simulink model "ur_ros"  (R2024a)
settings: Solver=FixedStepAuto  StartTime=0.0  StopTime=inf  RelTol=1e-3
undefined symbols (not defined in the file): duration, effort, index, joint1, joint2, joint3, joint4, joint5, joint6, joint_name, model_name, q0, Ts, ur
libraries: robotgazebolib x26, robotmaniplib x3, slpidlib x1
settings Model: Creator=26092  LastModifiedBy=26092

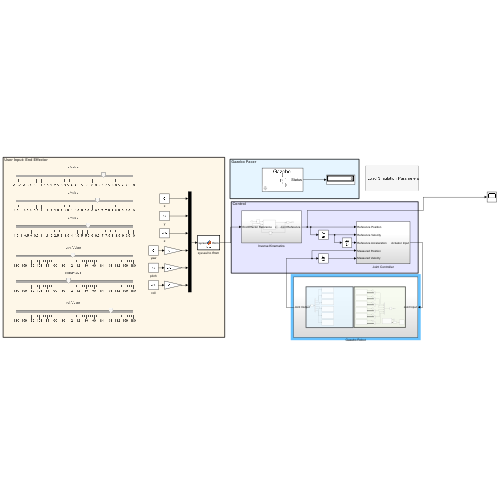
[thumbnail: Simulink's stored preview of the top-level diagram]
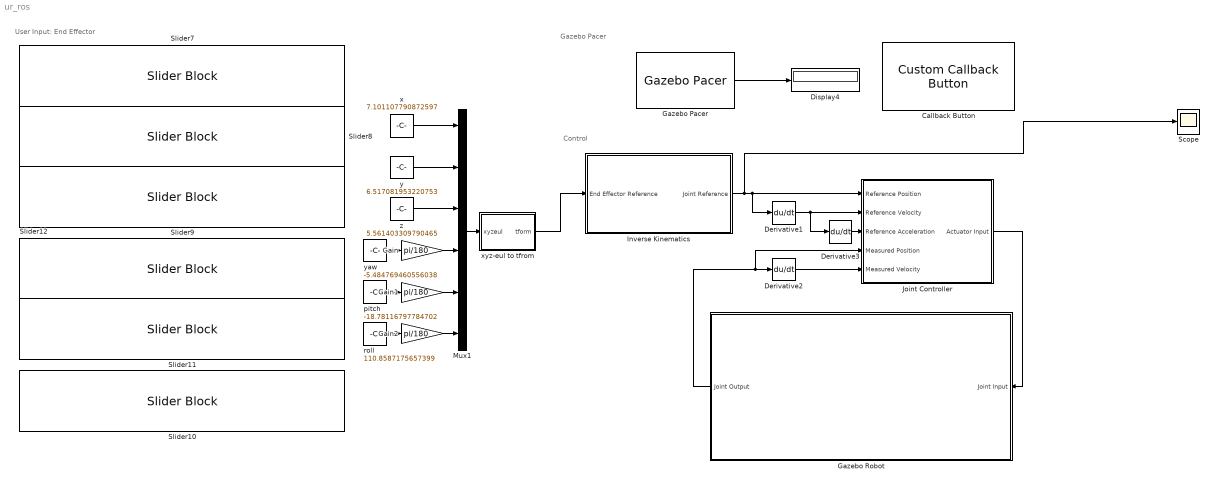
== system ur_ros ==
  note: User Input: End Effector
  note: Control
  note: Gazebo Pacer
  Callback Button : CustomCallbackButton  Configuration="{\"components\":[{\"name\":\"BackgroundImageComponent\",\"settings\":{\"image\":{\"size\":[0,0],\"src\":\"default\",\"srcOrientation\":\"Right\"},\"position\":[0,0,1,1]}},{\"name\":\"ButtonStateComponent\",\"settings\":{\"buttonType\":\"momentary\",\"clickFcn\":\" % Set sample times\\n  Ts = 0.01;\\n  Ts_trajectory = 0.05;\\n\\n  % Load the robot - 使用自定义URDF模型\\n  robot = importrobot('ur.urdf');\\n  robot.Gravity = [0 0 -9.81];\\n  robot.DataFormat = 'column';\\n\\n  % 显示机器人信息确认加载\\n  showdetails(robot);\\n  disp('机器人模型 robot 已成功加载！');\\n\\n  % IK initial guess\\n  q0 = [0 -70 140 0 0 0]' * pi\\/180;\\n\\n  % Custom bus objects\\n  load('custom_busobjects_basic');\",\"onValue\":1,\"position\":[0,0,1,1],\"pressDelay\":\"500\",\"pressFcn\":\"\",\"repeatInterval\":\"0\",\"states\":[{\"horizontalAlignment\":\"center\",\"image\":{\"position\":[0,0,1,1],\"size\":[1,1],\"src\":\"default\",\"srcOrientation\":\"Right\"},\"label\":{\"color\":[0.01176470588,0.01176470588,0.01176470588,1],\"icon\":{\"size\":[0,0],\"src\":\"default\",\"srcOrientation\":\"Right\"},\"iconPlacement\":\"left\",\"opacity\":1,\"show\":true,\"text\":{\"content\":\"Load Simulation Parameters\",\"font\":\"Helvetica\",\"fontSize\":15}},\"labelOffset\":[0,0],\"verticalAlignment\":\"middle\"},{\"horizontalAlignment\":\"center\",\"image\":{\"position\":[0,0,1,1],\"size\":[1,1],\"src\":\"default\",\"srcOrientation\":\"Right\"},\"label\":{\"color\":[0.01176470588,0.01176470588,0.01176470588,1],\"icon\":{\"size\":[0,0],\"src\":\"default\",\"srcOrientation\":\"Right\"},\"iconPlacement\":\"left\",\"opacity\":1,\"show\":true,\"text\":{\"content\":\"Load Simulation Parameters\",\"font\":\"Helvetica\",\"fontSize\":15}},\"labelOffset\":[0,0],\"verticalAlignment\":\"middle\"},{\"horizontalAlignment\":\"center\",\"image\":{\"position\":[0,0,1,1],\"size\":[1,1],\"src\":\"default\",\"srcOrientation\":\"Right\"},\"label\":{\"color\":[0.01176470588,0.01176470588,0.01176470588,1],\"icon\":{\"size\":[0,0],\"src\":\"default\",\"srcOrientation\":\"Right\"},\"iconPlacement\":\"left\",\"opacity\":1,\"show\":true,\"text\":{\"content\":\"Load Simulation Parameters\",\"font\":\"Helvetica\",\"fontSize\":15}},\"labelOffset\":[0,0],\"verticalAlignment\":\"middle\"},{\"horizontalAlignment\":\"center\",\"image\":{\"position\":[0,0,1,1],\"size\":[1,1],\"src\":\"default\",\"srcOrientation\":\"Right\"},\"label\":{\"color\":[0.01176470588,0.01176470588,0.01176470588,1],\"icon\":{\"size\":[0,0],\"src\":\"default\",\"srcOrientation\":\"Right\"},\"iconPlacement\":\"left\",\"opacity\":1,\"show\":true,\"text\":{\"content\":\"Load Simulation Parameters\",\"font\":\"Helvetica\",\"fontSize\":15}},\"labelOffset\":[0,0],\"verticalAlignment\":\"middle\"}]}},{\"name\":\"ForegroundImageComponent\",\"settings\":{\"image\":{\"size\":[0,0],\"src\":\"default\",\"srcOrientation\":\"Right\"},\"isForeground\":1,\"position\":[0,0,1,1]}}],\"settings\":{\"BindingType\":\"standalone\",\"backgroundColor\":[244,244,244,1],\"backgroundOffset\":0.2,\"backgroundOpacity\":1,\"fixedAspectRatio\":\"off\",\"foregroundColor\":[0.01176470588,0.01176470588,0.01176470588,1],\"migratedFromLegacy\":true,\"useBackgroundColor\":true,\"variant\":\"callback\",\"version\":\"R2023a\"},\"type\":\"Button\"}"  CustomBackgroundColor="{\"color\":[0.9568627451,0.9568627451,0.9568627451],\"show\":true}"
  Derivative1 : Derivative
  Derivative2 : Derivative
  Derivative3 : Derivative
  Display4 : Display
  Gain : Gain  Gain=pi/180
  Gain1 : Gain  Gain=pi/180
  Gain2 : Gain  Gain=pi/180
  Gazebo Pacer : robotgazebolib/Gazebo Pacer  ResetBehavior=Reset Gazebo simulation time  SampleTime=Ts
  Gazebo Robot : Subsystem
  Inverse Kinematics : Subsystem
  Joint Controller : Subsystem  VariantControl=actuator_type == 2
  Mux1 : Mux  Inputs=6
  Scope : Scope
  Slider10 : SliderBlock  ScaleMin=-180  ScaleMax=180
  Slider11 : SliderBlock  ScaleMin=-180  ScaleMax=180
  Slider12 : SliderBlock  ScaleMin=-180  ScaleMax=180
  Slider7 : SliderBlock  ScaleMin=-1.5  ScaleMax=10
  Slider8 : SliderBlock  ScaleMin=-1.5  ScaleMax=10
  Slider9 : SliderBlock  ScaleMin=-1.5  ScaleMax=10
  pitch : Constant  InitFcn=set_param(gcb,'Value','-70')  Value=-18.78116797784702
  roll : Constant  InitFcn=set_param(gcb,'Value','90')  Value=110.8587175657399
  x : Constant  InitFcn=set_param(gcb,'Value','0.3')  Value=7.101107790872597
  xyz-eul to tfrom : MATLAB Function  TreatAsAtomicUnit=on
  y : Constant  InitFcn=set_param(gcb,'Value','0.25')  Value=6.517081953220753
  yaw : Constant  InitFcn=set_param(gcb,'Value','180')  Value=-5.484769460556038
  z : Constant  InitFcn=set_param(gcb,'Value','0.125')  Value=5.561403309790465
  wires:
  Gazebo Robot/1(Joint Output) -> Joint Controller/4(Measured Position), Derivative2/1
  roll/1 -> Gain2/1
  Joint Controller/1(Actuator Input) -> Gazebo Robot/1(Joint Input)
  Gain/1 -> Mux1/4
  z/1 -> Mux1/3
  Inverse Kinematics/1(Joint Reference) -> Scope/1, Derivative1/1, Joint Controller/1(Reference Position)
  Derivative1/1 -> Joint Controller/2(Reference Velocity), Derivative3/1
  Derivative2/1 -> Joint Controller/5(Measured Velocity)
  Derivative3/1 -> Joint Controller/3(Reference Acceleration)
  Mux1/1 -> xyz-eul to tfrom/1(xyzeul)
  Gain1/1 -> Mux1/5
  yaw/1 -> Gain/1
  xyz-eul to tfrom/1(tform) -> Inverse Kinematics/1(End Effector Reference)
  x/1 -> Mux1/1
  pitch/1 -> Gain1/1
  y/1 -> Mux1/2
  Gazebo Pacer/1 -> Display4/1
  Gain2/1 -> Mux1/6

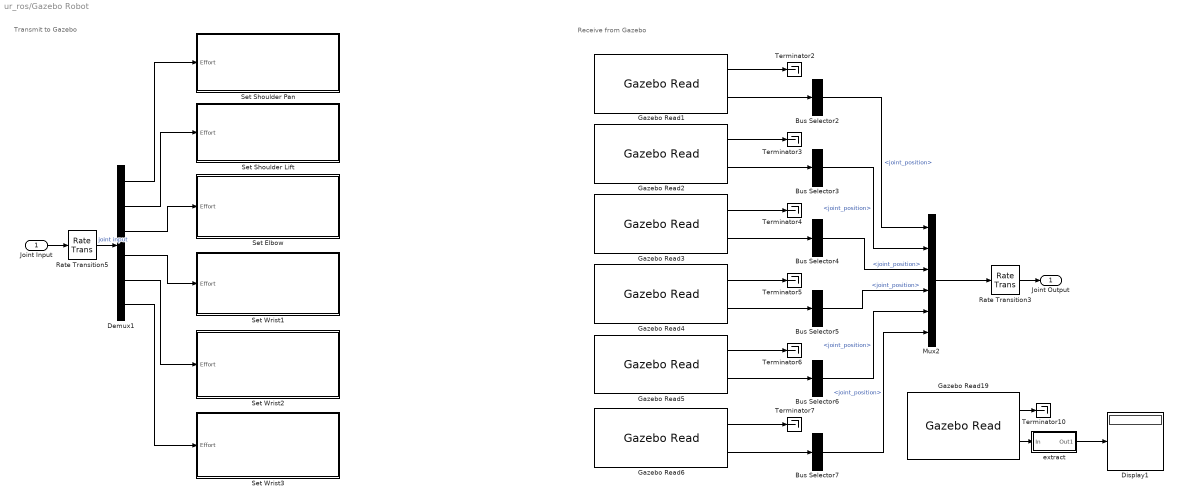
== system ur_ros/Gazebo Robot ==
  note: Receive from Gazebo
  note: Transmit to Gazebo
  Joint Input : Inport
  Bus Selector{2..7} (6 alike) : BusSelector  OutputSignals=joint_position
  Demux1 : Demux  Outputs=6
  Display1 : Display
  Gazebo Read1 : robotgazebolib/Gazebo Read  topicSource=From Gazebo  topic=/gazebo/ground_truth/joint_state/ur/joint1  messageType=gazebo_msgs/JointState_fixed_1  sampleTime=Ts  fixedAxisBusStatus=on  jointAxisCount=1
  Gazebo Read19 : robotgazebolib/Gazebo Read  topicSource=From Gazebo  topic=/gazebo/ground_truth/world_pose/redBox/link  messageType=gazebo_msgs/Pose  sampleTime=Ts  fixedAxisBusStatus=off  jointAxisCount=2
  Gazebo Read2 : robotgazebolib/Gazebo Read  topicSource=From Gazebo  topic=/gazebo/ground_truth/joint_state/ur/joint2  messageType=gazebo_msgs/JointState_fixed_1  sampleTime=Ts  fixedAxisBusStatus=on  jointAxisCount=1
  Gazebo Read3 : robotgazebolib/Gazebo Read  topicSource=From Gazebo  topic=/gazebo/ground_truth/joint_state/ur/joint3  messageType=gazebo_msgs/JointState_fixed_1  sampleTime=Ts  fixedAxisBusStatus=on  jointAxisCount=1
  Gazebo Read4 : robotgazebolib/Gazebo Read  topicSource=From Gazebo  topic=/gazebo/ground_truth/joint_state/ur/joint4  messageType=gazebo_msgs/JointState_fixed_1  sampleTime=Ts  fixedAxisBusStatus=on  jointAxisCount=1
  Gazebo Read5 : robotgazebolib/Gazebo Read  topicSource=From Gazebo  topic=/gazebo/ground_truth/joint_state/ur/joint5  messageType=gazebo_msgs/JointState_fixed_1  sampleTime=Ts  fixedAxisBusStatus=on  jointAxisCount=1
  Gazebo Read6 : robotgazebolib/Gazebo Read  topicSource=From Gazebo  topic=/gazebo/ground_truth/joint_state/ur/joint6  messageType=gazebo_msgs/JointState_fixed_1  sampleTime=Ts  fixedAxisBusStatus=on  jointAxisCount=1
  Mux2 : Mux  Inputs=6
  Rate Transition3 : RateTransition  OutPortSampleTime=Ts
  Rate Transition5 : RateTransition  OutPortSampleTime=Ts
  Set Elbow : Subsystem
  Set Shoulder Lift : Subsystem
  Set Shoulder Pan : Subsystem
  Set Wrist1 : Subsystem
  Set Wrist2 : Subsystem
  Set Wrist3 : Subsystem
  Terminator{2..7,10} (7 alike) : Terminator
  extract : Subsystem
  Joint Output : Outport
  wires:
  Mux2/1 -> Rate Transition3/1
  Bus Selector4/1 -> Mux2/3  "<joint_position>"
  Demux1/2 -> Set Shoulder Lift/1(Effort)
  Bus Selector3/1 -> Mux2/2  "<joint_position>"
  Bus Selector6/1 -> Mux2/5  "<joint_position>"
  Gazebo Read5/1 -> Terminator6/1
  Gazebo Read1/2 -> Bus Selector2/1
  Gazebo Read1/1 -> Terminator2/1
  Bus Selector7/1 -> Mux2/6  "<joint_position>"
  Bus Selector5/1 -> Mux2/4  "<joint_position>"
  Gazebo Read6/2 -> Bus Selector7/1
  Gazebo Read2/2 -> Bus Selector3/1
  Gazebo Read5/2 -> Bus Selector6/1
  Gazebo Read2/1 -> Terminator3/1
  Gazebo Read4/2 -> Bus Selector5/1
  Gazebo Read4/1 -> Terminator5/1
  Gazebo Read19/2 -> extract/1(In)
  Joint Input/1 -> Rate Transition5/1
  Bus Selector2/1 -> Mux2/1  "<joint_position>"
  Gazebo Read19/1 -> Terminator10/1
  Demux1/5 -> Set Wrist2/1(Effort)
  Demux1/3 -> Set Elbow/1(Effort)
  Gazebo Read3/1 -> Terminator4/1
  extract/1(Out1) -> Display1/1
  Gazebo Read3/2 -> Bus Selector4/1
  Gazebo Read6/1 -> Terminator7/1
  Rate Transition3/1 -> Joint Output/1
  Rate Transition5/1 -> Demux1/1  "joint input"
  Demux1/4 -> Set Wrist1/1(Effort)
  Demux1/6 -> Set Wrist3/1(Effort)
  Demux1/1 -> Set Shoulder Pan/1(Effort)

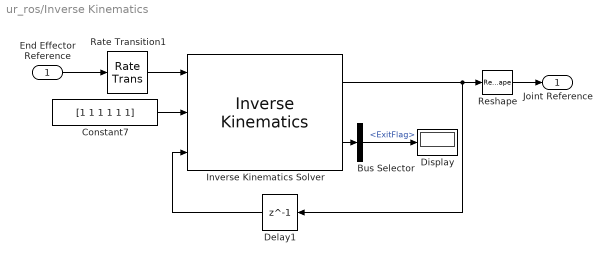
== system ur_ros/Inverse Kinematics ==
  End Effector Reference : Inport
  Bus Selector : BusSelector  OutputSignals=ExitFlag
  Constant7 : Constant  Value=[1 1 1 1 1 1]  SampleTime=-1
  Delay1 : Delay  DelayLength=1  InitialCondition=q0
  Display : Display
  Inverse Kinematics Solver : robotmaniplib/Inverse Kinematics  RigidBodyTree=robot  EndEffector=link6  ShowInfo=on  SolverName=BFGS Gradient Projection  EnforceJointLimits=on  MaxIterations=150  MaxTime=1  GradientTolerance=1e-7  SolutionTolerance=1e-5  StepTolerance=1e-14  ErrorChangeTolerance=1e-8  UseErrorDamping=on  DampingBias=0.0025  SimulateUsing=Interpreted execution
  Rate Transition1 : RateTransition  OutPortSampleTime=Ts_trajectory
  Reshape : Reshape
  Joint Reference : Outport
  wires:
  Inverse Kinematics Solver/1 -> Delay1/1, Reshape/1
  End Effector Reference/1 -> Rate Transition1/1
  Delay1/1 -> Inverse Kinematics Solver/3
  Constant7/1 -> Inverse Kinematics Solver/2
  Inverse Kinematics Solver/2 -> Bus Selector/1
  Reshape/1 -> Joint Reference/1
  Rate Transition1/1 -> Inverse Kinematics Solver/1
  Bus Selector/1 -> Display/1  "<ExitFlag>"

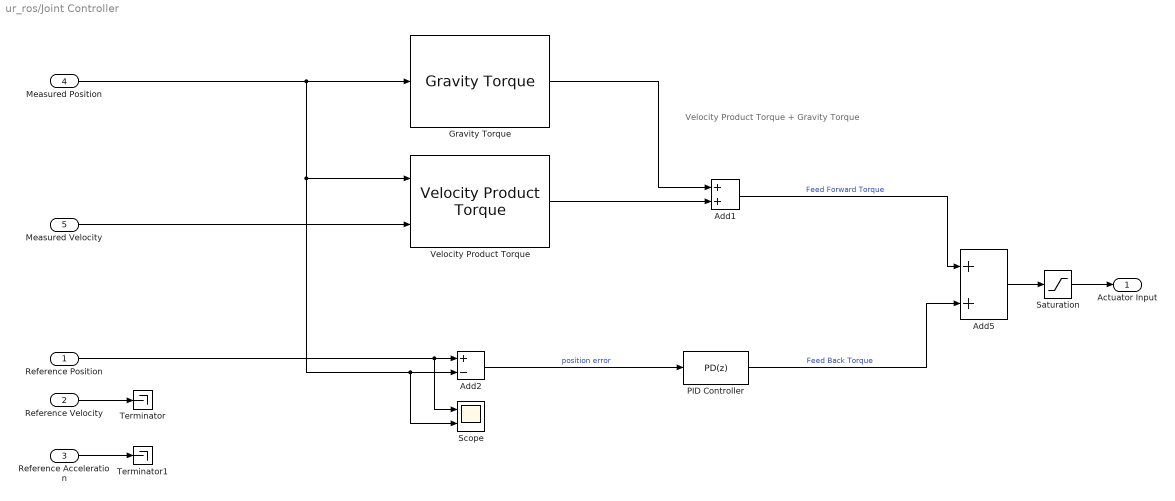
== system ur_ros/Joint Controller ==
  note: Velocity Product Torque + Gravity Torque
  Reference Position : Inport
  Reference Velocity : Inport  Port=2
  Reference Acceleration : Inport  Port=3
  Measured Position : Inport  Port=4
  Measured Velocity : Inport  Port=5
  Add1 : Sum
  Add2 : Sum  Inputs=+-
  Add5 : Sum
  Gravity Torque : robotmaniplib/Gravity Torque  RigidBodyTree=robot  SimulateUsing=Interpreted execution
  PID Controller : slpidlib/PID Controller  Controller=PD  Form=Parallel  TimeDomain=Discrete-time  UseExternalTs=off  SampleTime=-1  IntegratorMethod=Forward Euler  FilterMethod=Forward Euler  ControllerParametersSource=internal  P=[128 128 128 16 4 0.1]  I=[0 0 0 0 0 0]  UseKiTs=off  D=[40 32 32 1.6 0.4 0.01]  UseExternalDerivativeSource=off  N=100  UseFilter=on  TunerSelectOption=Transfer Function Based (PID Tuner App)  ZeroCross=off  InitialConditionSource=internal  InitialConditionForIntegrator=0  InitialConditionForFilter=0  DifferentiatorICPrevScaledInput=0  ExternalReset=none  TrackingMode=off  Kt=1  LimitOutput=off  SatLimitsSource=internal  UpperSaturationLimit=inf  LowerSaturationLimit=-inf  LinearizeAsGain=on  AntiWindupMode=none  Kb=1  LimitIntegrator=off  UpperIntegratorSaturationLimit=inf  LowerIntegratorSaturationLimit=-inf  POutMin=[]  POutMax=[]  IOutMin=[]  IOutMax=[]  DOutMin=[]  DOutMax=[]  NOutMin=[]  NOutMax=[]  SumOutMin=[]  SumOutMax=[]  SaturationOutMin=[]  SaturationOutMax=[]  PParamMin=[]  PParamMax=[]  IParamMin=[]  IParamMax=[]  DParamMin=[]  DParamMax=[]  NParamMin=[]  NParamMax=[]  KbParamMin=[]  KbParamMax=[]  KtParamMin=[]  KtParamMax=[]  KbOutMin=[]  KbOutMax=[]  KtOutMin=[]  KtOutMax=[]  IntegratorOutMin=[]  IntegratorOutMax=[]  FilterOutMin=[]  FilterOutMax=[]  SumI1OutMin=[]  SumI1OutMax=[]  SumI2OutMin=[]  SumI2OutMax=[]  SumI3OutMin=[]  SumI3OutMax=[]  SumI4OutMin=[]  SumI4OutMax=[]  SumDOutMin=[]  SumDOutMax=[]  DifferentiatorOutMin=[]  DifferentiatorOutMax=[]  FilterDiffOutCoefMin=[]  FilterDiffOutCoefMax=[]  ReciprocalOutMin=[]  ReciprocalOutMax=[]  SumDenOutMin=[]  SumDenOutMax=[]  SumNumOutMin=[]  SumNumOutMax=[]  DivideOutMin=[]  DivideOutMax=[]  UdiffTsProdOutMin=[]  UdiffTsProdOutMax=[]  NTsProdOutMin=[]  NTsProdOutMax=[]  UintegralTsProdOutMin=[]  UintegralTsProdOutMax=[]  UngainTsProdOutMin=[]  UngainTsProdOutMax=[]  ClampingZeroOutDataTypeStr=Inherit: Inherit via back propagation  ClampingZeroOutMin=[]  ClampingZeroOutMax=[]  FilterDenConstantOutDataTypeStr=Inherit: Inherit via back propagation  FilterDenConstantOutMin=[]  FilterDenConstantOutMax=[]  PCopyOutDataTypeStr=Inherit: Inherit via back propagation  PCopyOutMin=[]  PCopyOutMax=[]  NCopyOutDataTypeStr=Inherit: Inherit via back propagation  NCopyOutMin=[]  NCopyOutMax=[]  IntegratorContinuousStateAttributes=''  IntegratorStateMustResolveToSignalObject=off  IntegratorRTWStateStorageClass=Auto  FilterContinuousStateAttributes=''  FilterStateMustResolveToSignalObject=off  FilterRTWStateStorageClass=Auto  ParallelPVariant=InternalParameters  IdealPVariant=Disabled  IVariant=Disabled  DVariant=InternalParameters  IntegratorVariant=Disabled  SatVariant=Disabled  AWVariant=Disabled  PCopyVariant=Disabled  TRVariant=Disabled  FdbkBlocksVariant=Forward  IdealPFdbkVariant=Disabled  SatFdbkVariant=Disabled  DerivativeFilterVariant=ForwardEulerFilter  NVariant=InternalParameters  NCopyVariant=Disabled  FilterICVariant=InternalICsFilter  IntegratorICVariant=Disabled  ExternalResetVariant=Disabled  TRSumVariant=Passthrough  SumFdbkVariant=Disabled  SumVariant=Sum_PD  TsampFilterVariant=InternalTs  TsampNgainVariant=Passthrough  TsampIntegralVariant=Disabled_SignalSpec  ExternalSaturationOutDataTypeStr=Inherit: Same as second input  DerivativeSourceVariant=ErrorSignal
  Saturation : Saturate  UpperLimit=[330 330 150 54 54 54]  LowerLimit=[-330 -330 -150 -54 -54 -54]
  Scope : Scope  NumInputPorts=2
  Terminator : Terminator
  Terminator1 : Terminator
  Velocity Product Torque : robotmaniplib/Velocity Product Torque  RigidBodyTree=robot  SimulateUsing=Interpreted execution
  Actuator Input : Outport  VectorParamsAs1DForOutWhenUnconnected=off
  wires:
  Reference Position/1 -> Scope/1, Add2/1
  Measured Position/1 -> Gravity Torque/1, Scope/2, Add2/2, Velocity Product Torque/1
  Measured Velocity/1 -> Velocity Product Torque/2
  Add5/1 -> Saturation/1
  Add1/1 -> Add5/1  "Feed Forward Torque"
  Gravity Torque/1 -> Add1/1
  Velocity Product Torque/1 -> Add1/2
  Saturation/1 -> Actuator Input/1
  Add2/1 -> PID Controller/1  "position error"
  PID Controller/1 -> Add5/2  "Feed Back Torque"
  Reference Velocity/1 -> Terminator/1
  Reference Acceleration/1 -> Terminator1/1

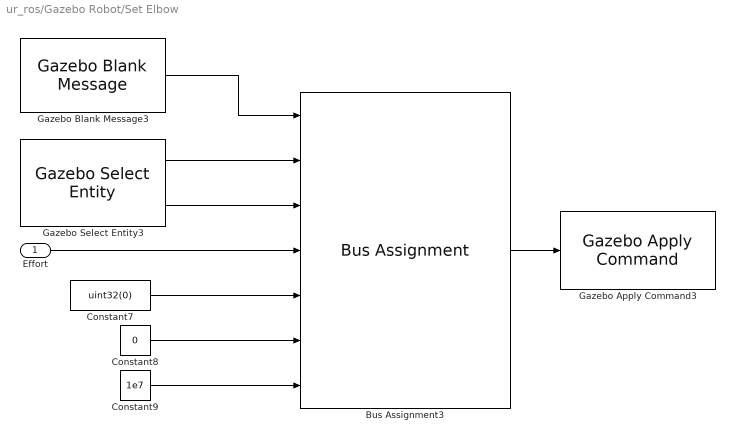
== system ur_ros/Gazebo Robot/Set Elbow ==
  Effort : Inport
  Bus Assignment3 : BusAssignment  AssignedSignals=model_name,joint_name,effort,index,duration.seconds,duration.nano_seconds
  Constant7 : Constant  Value=uint32(0)
  Constant8 : Constant  Value=0
  Constant9 : Constant  Value=1e7
  Gazebo Apply Command3 : robotgazebolib/Gazebo Apply Command  cmdType=ApplyJointTorque  sampleTime=Ts
  Gazebo Blank Message3 : robotgazebolib/Gazebo Blank Message  msgType=ApplyJointTorque  sampleTime=Ts  busName='Gazebo_SL_Bus_gazebo_msgs_ApplyJointTorque'
  Gazebo Select Entity3 : robotgazebolib/Gazebo Select Entity  modelElemName=ur/joint3  outputArraySize=128  OutputLabel=Joint  SelectType=Joint
  wires:
  Gazebo Select Entity3/1 -> Bus Assignment3/2
  Bus Assignment3/1 -> Gazebo Apply Command3/1
  Constant8/1 -> Bus Assignment3/6
  Constant9/1 -> Bus Assignment3/7
  Gazebo Blank Message3/1 -> Bus Assignment3/1
  Gazebo Select Entity3/2 -> Bus Assignment3/3
  Constant7/1 -> Bus Assignment3/5
  Effort/1 -> Bus Assignment3/4

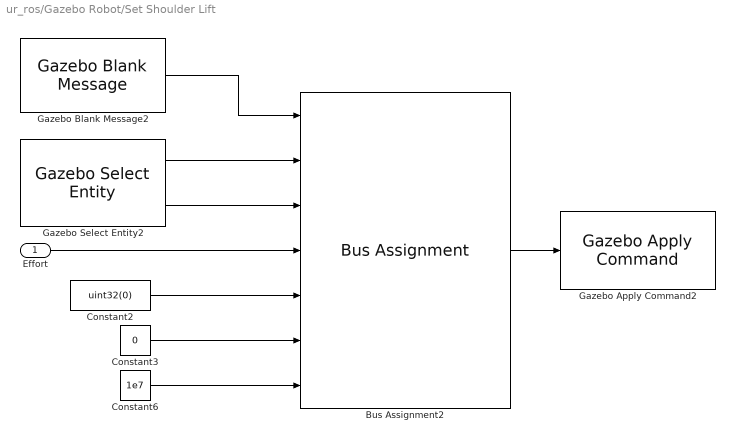
== system ur_ros/Gazebo Robot/Set Shoulder Lift ==
  Effort : Inport
  Bus Assignment2 : BusAssignment  AssignedSignals=model_name,joint_name,effort,index,duration.seconds,duration.nano_seconds
  Constant2 : Constant  Value=uint32(0)
  Constant3 : Constant  Value=0
  Constant6 : Constant  Value=1e7
  Gazebo Apply Command2 : robotgazebolib/Gazebo Apply Command  cmdType=ApplyJointTorque  sampleTime=Ts
  Gazebo Blank Message2 : robotgazebolib/Gazebo Blank Message  msgType=ApplyJointTorque  sampleTime=Ts  busName='Gazebo_SL_Bus_gazebo_msgs_ApplyJointTorque'
  Gazebo Select Entity2 : robotgazebolib/Gazebo Select Entity  modelElemName=ur/joint2  outputArraySize=128  OutputLabel=Joint  SelectType=Joint
  wires:
  Gazebo Select Entity2/1 -> Bus Assignment2/2
  Constant6/1 -> Bus Assignment2/7
  Gazebo Select Entity2/2 -> Bus Assignment2/3
  Gazebo Blank Message2/1 -> Bus Assignment2/1
  Bus Assignment2/1 -> Gazebo Apply Command2/1
  Constant3/1 -> Bus Assignment2/6
  Effort/1 -> Bus Assignment2/4
  Constant2/1 -> Bus Assignment2/5

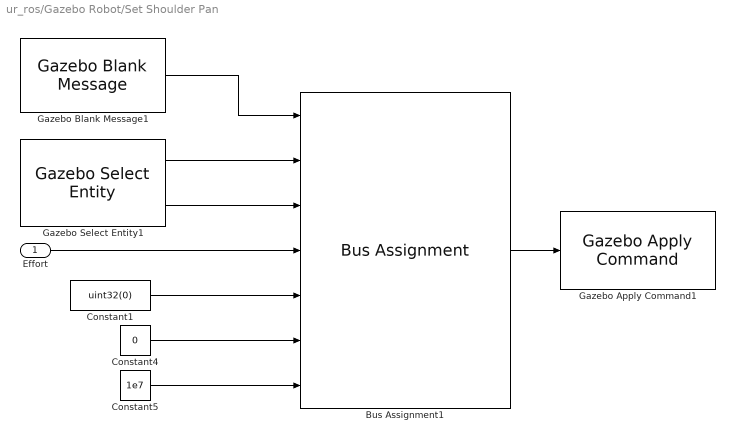
== system ur_ros/Gazebo Robot/Set Shoulder Pan ==
  Effort : Inport
  Bus Assignment1 : BusAssignment  AssignedSignals=model_name,joint_name,effort,index,duration.seconds,duration.nano_seconds
  Constant1 : Constant  Value=uint32(0)
  Constant4 : Constant  Value=0
  Constant5 : Constant  Value=1e7
  Gazebo Apply Command1 : robotgazebolib/Gazebo Apply Command  cmdType=ApplyJointTorque  sampleTime=Ts
  Gazebo Blank Message1 : robotgazebolib/Gazebo Blank Message  msgType=ApplyJointTorque  sampleTime=Ts  busName='Gazebo_SL_Bus_gazebo_msgs_ApplyJointTorque'
  Gazebo Select Entity1 : robotgazebolib/Gazebo Select Entity  modelElemName=ur/joint1  outputArraySize=128  OutputLabel=Joint  SelectType=Joint
  wires:
  Constant1/1 -> Bus Assignment1/5
  Effort/1 -> Bus Assignment1/4
  Bus Assignment1/1 -> Gazebo Apply Command1/1
  Gazebo Select Entity1/1 -> Bus Assignment1/2
  Constant4/1 -> Bus Assignment1/6
  Gazebo Blank Message1/1 -> Bus Assignment1/1
  Gazebo Select Entity1/2 -> Bus Assignment1/3
  Constant5/1 -> Bus Assignment1/7

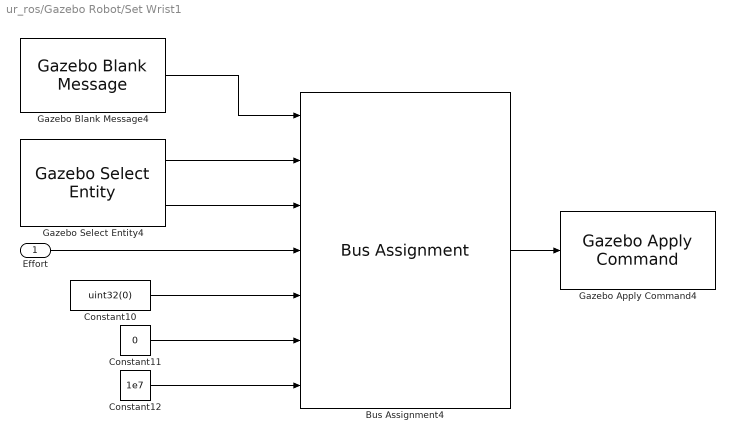
== system ur_ros/Gazebo Robot/Set Wrist1 ==
  Effort : Inport
  Bus Assignment4 : BusAssignment  AssignedSignals=model_name,joint_name,effort,index,duration.seconds,duration.nano_seconds
  Constant10 : Constant  Value=uint32(0)
  Constant11 : Constant  Value=0
  Constant12 : Constant  Value=1e7
  Gazebo Apply Command4 : robotgazebolib/Gazebo Apply Command  cmdType=ApplyJointTorque  sampleTime=Ts
  Gazebo Blank Message4 : robotgazebolib/Gazebo Blank Message  msgType=ApplyJointTorque  sampleTime=Ts  busName='Gazebo_SL_Bus_gazebo_msgs_ApplyJointTorque'
  Gazebo Select Entity4 : robotgazebolib/Gazebo Select Entity  modelElemName=ur/joint4  outputArraySize=128  OutputLabel=Joint  SelectType=Joint
  wires:
  Bus Assignment4/1 -> Gazebo Apply Command4/1
  Constant12/1 -> Bus Assignment4/7
  Effort/1 -> Bus Assignment4/4
  Constant11/1 -> Bus Assignment4/6
  Gazebo Select Entity4/2 -> Bus Assignment4/3
  Constant10/1 -> Bus Assignment4/5
  Gazebo Select Entity4/1 -> Bus Assignment4/2
  Gazebo Blank Message4/1 -> Bus Assignment4/1

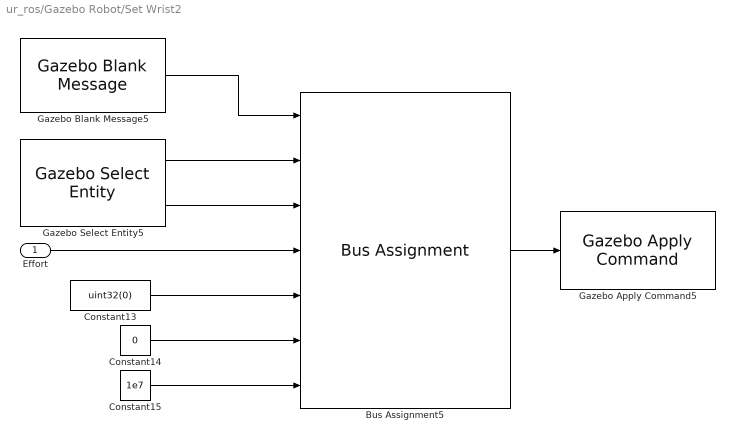
== system ur_ros/Gazebo Robot/Set Wrist2 ==
  Effort : Inport
  Bus Assignment5 : BusAssignment  AssignedSignals=model_name,joint_name,effort,index,duration.seconds,duration.nano_seconds
  Constant13 : Constant  Value=uint32(0)
  Constant14 : Constant  Value=0
  Constant15 : Constant  Value=1e7
  Gazebo Apply Command5 : robotgazebolib/Gazebo Apply Command  cmdType=ApplyJointTorque  sampleTime=Ts
  Gazebo Blank Message5 : robotgazebolib/Gazebo Blank Message  msgType=ApplyJointTorque  sampleTime=Ts  busName='Gazebo_SL_Bus_gazebo_msgs_ApplyJointTorque'
  Gazebo Select Entity5 : robotgazebolib/Gazebo Select Entity  modelElemName=ur/joint5  outputArraySize=128  OutputLabel=Joint  SelectType=Joint
  wires:
  Gazebo Select Entity5/2 -> Bus Assignment5/3
  Gazebo Select Entity5/1 -> Bus Assignment5/2
  Constant13/1 -> Bus Assignment5/5
  Constant14/1 -> Bus Assignment5/6
  Constant15/1 -> Bus Assignment5/7
  Effort/1 -> Bus Assignment5/4
  Gazebo Blank Message5/1 -> Bus Assignment5/1
  Bus Assignment5/1 -> Gazebo Apply Command5/1

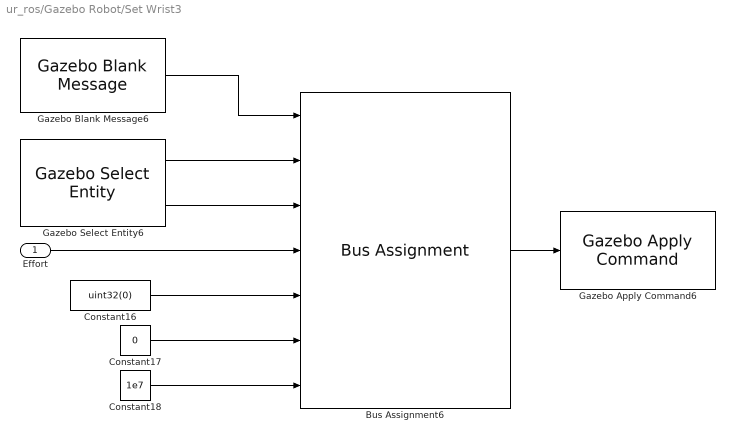
== system ur_ros/Gazebo Robot/Set Wrist3 ==
  Effort : Inport
  Bus Assignment6 : BusAssignment  AssignedSignals=model_name,joint_name,effort,index,duration.seconds,duration.nano_seconds
  Constant16 : Constant  Value=uint32(0)
  Constant17 : Constant  Value=0
  Constant18 : Constant  Value=1e7
  Gazebo Apply Command6 : robotgazebolib/Gazebo Apply Command  cmdType=ApplyJointTorque  sampleTime=Ts
  Gazebo Blank Message6 : robotgazebolib/Gazebo Blank Message  msgType=ApplyJointTorque  sampleTime=Ts  busName='Gazebo_SL_Bus_gazebo_msgs_ApplyJointTorque'
  Gazebo Select Entity6 : robotgazebolib/Gazebo Select Entity  modelElemName=ur/joint6  outputArraySize=128  OutputLabel=Joint  SelectType=Joint
  wires:
  Bus Assignment6/1 -> Gazebo Apply Command6/1
  Gazebo Blank Message6/1 -> Bus Assignment6/1
  Gazebo Select Entity6/1 -> Bus Assignment6/2
  Constant16/1 -> Bus Assignment6/5
  Gazebo Select Entity6/2 -> Bus Assignment6/3
  Constant17/1 -> Bus Assignment6/6
  Constant18/1 -> Bus Assignment6/7
  Effort/1 -> Bus Assignment6/4

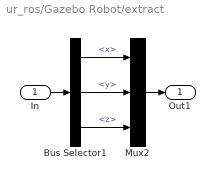
== system ur_ros/Gazebo Robot/extract ==
  In : Inport
  Bus Selector1 : BusSelector  OutputSignals=position.x,position.y,position.z
  Mux2 : Mux  Inputs=3
  Out1 : Outport
  wires:
  In/1 -> Bus Selector1/1
  Bus Selector1/1 -> Mux2/1  "<x>"
  Mux2/1 -> Out1/1
  Bus Selector1/2 -> Mux2/2  "<y>"
  Bus Selector1/3 -> Mux2/3  "<z>"

== matlab function ur_ros/xyz-eul to tfrom ==
  data: xyzeul input; tform output
function tform = fcn(xyzeul)

targetmat = eul2tform(xyzeul(4:6)'); 
targetmat(1:3,end) = xyzeul(1:3); 
tform = targetmat;
